simulink model "case3_sensitivity"  (Simulink 6.6)
settings: Solver=ode45  StartTime=0.0  StopTime=36  RelTol=1e-3
undefined symbols (not defined in the file or in its folder): sigbuilder_block
settings Model: Creator=MXKana  LastModifiedBy=mxkana

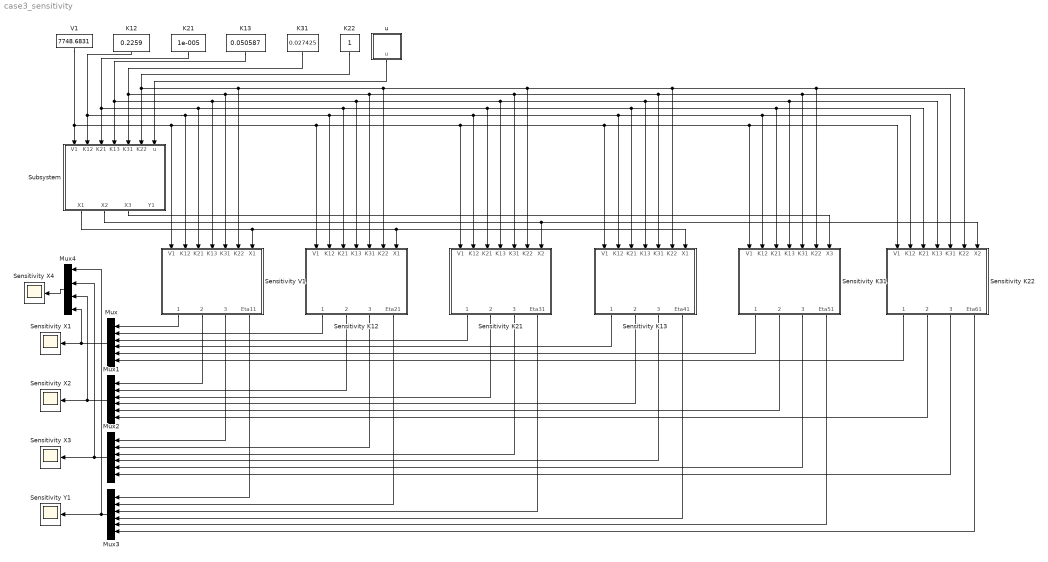
== system case3_sensitivity ==
  K12 : Constant  Orientation=down  Value=0.2259
  K13 : Constant  Orientation=down  Value=0.050587
  K21 : Constant  Orientation=down  Value=1e-005
  K22 : Constant  Orientation=down
  K31 : Constant  Orientation=down  Value=0.027425
  Mux{,1..3} (4 alike) : Mux  Orientation=left  Inputs=6
  Mux4 : Mux  Orientation=left
  Sensitivity K12 : Subsystem  Orientation=down
  Sensitivity K13 : Subsystem  Orientation=down
  Sensitivity K21 : Subsystem  Orientation=down
  Sensitivity K22 : Subsystem  Orientation=down
  Sensitivity K31 : Subsystem  Orientation=down
  Sensitivity V1 : Subsystem  Orientation=down
  Sensitivity X{1..4} (4 alike) : Scope
      Sensitivity X3 settings: SaveName=ScopeData2
      Sensitivity X4 settings: SaveName=ScopeData4
  Sensitivity Y1 : Scope
      settings: SaveName=ScopeData5
  Subsystem : Subsystem  Orientation=down
  V1 : Constant  Orientation=down  Value=7748.6831
  u : Subsystem  Tag=STV Subsys  Orientation=down  LoadFcn=sigbuilder_block('load');  StartFcn=sigbuilder_block('start');  StopFcn=sigbuilder_block('stop');  ClipboardFcn=sigbuilder_block('clipboard');  mask(Sigbuilder block){}
      mask help: Sigbuilder GUI
      mask init:
      | if ~strcmp(get_param(bdroot(gcbh),'SimulationStatus'),'stopped') tuvar = sigbuilder_block('maskInit'); end
      settings: CopyFcn=sigbuilder_block('copy');  DeleteFcn=sigbuilder_block('delete');  ModelCloseFcn=sigbuilder_block('modelClose');  PreSaveFcn=sigbuilder_block('preSave');  NameChangeFcn=sigbuilder_block('namechange');  OpenFcn=sigbuilder_block('open',[406.5 183 550.5 363.75 ]);  CloseFcn=sigbuilder_block('close');
      mask Display: plot(0,0,100,100,[10,10,40,40,10],[80,20,20,80,80],[40,10],[50,50], [40,27,10],[65,72,56],[40,25,25,10],[28,28,43,43]);
  wires:
  V1/1 -> Subsystem/1(V1), Sensitivity V1/1(V1), Sensitivity K12/1(V1), Sensitivity K21/1(V1), Sensitivity K13/1(V1), Sensitivity K31/1(V1), Sensitivity K22/1(V1)
  K12/1 -> Subsystem/2(K12), Sensitivity V1/2(K12), Sensitivity K12/2(K12), Sensitivity K21/2(K12), Sensitivity K13/2(K12), Sensitivity K31/2(K12), Sensitivity K22/2(K12)
  K21/1 -> Subsystem/3(K21), Sensitivity V1/3(K21), Sensitivity K12/3(K21), Sensitivity K21/3(K21), Sensitivity K13/3(K21), Sensitivity K31/3(K21), Sensitivity K22/3(K21)
  K13/1 -> Subsystem/4(K13), Sensitivity V1/4(K13), Sensitivity K12/4(K13), Sensitivity K21/4(K13), Sensitivity K13/4(K13), Sensitivity K31/4(K13), Sensitivity K22/4(K13)
  K31/1 -> Subsystem/5(K31), Sensitivity V1/5(K31), Sensitivity K12/5(K31), Sensitivity K21/5(K31), Sensitivity K13/5(K31), Sensitivity K31/5(K31), Sensitivity K22/5(K31)
  K22/1 -> Subsystem/6(K22), Sensitivity V1/6(K22), Sensitivity K12/6(K22), Sensitivity K21/6(K22), Sensitivity K13/6(K22), Sensitivity K31/6(K22), Sensitivity K22/6(K22)
  u/1(u) -> Subsystem/7(u)
  Subsystem/1(X1) -> Sensitivity V1/7(X1), Sensitivity K12/7(X1), Sensitivity K13/7(X1)
  Subsystem/2(X2) -> Sensitivity K21/7(X2), Sensitivity K22/7(X2)
  Subsystem/3(X3) -> Sensitivity K31/7(X3)
  Sensitivity V1/1(Lambda11) -> Mux/1
  Sensitivity K12/1(Lambda21) -> Mux/2
  Sensitivity K21/1(Lambda31) -> Mux/3
  Sensitivity K13/1(Lambda41) -> Mux/4
  Sensitivity K31/1(Lambda51) -> Mux/5
  Sensitivity K22/1(Lambda61) -> Mux/6
  Mux/1 -> Sensitivity X1/1, Mux4/4
  Mux1/1 -> Sensitivity X2/1, Mux4/3
  Sensitivity V1/2(Lambda12) -> Mux1/1
  Sensitivity K12/2(Lambda22) -> Mux1/2
  Sensitivity K21/2(Lambda32) -> Mux1/3
  Sensitivity K13/2(Lambda42) -> Mux1/4
  Sensitivity K31/2(Lambda52) -> Mux1/5
  Sensitivity K22/2(Lambda62) -> Mux1/6
  Mux2/1 -> Sensitivity X3/1, Mux4/2
  Sensitivity V1/3(Lambda13) -> Mux2/1
  Sensitivity K12/3(Lambda23) -> Mux2/2
  Sensitivity K21/3(Lambda33) -> Mux2/3
  Sensitivity K13/3(Lambda43) -> Mux2/4
  Sensitivity K31/3(Lambda53) -> Mux2/5
  Sensitivity K22/3(Lambda63) -> Mux2/6
  Mux3/1 -> Mux4/1, Sensitivity Y1/1
  Sensitivity V1/4(Eta11) -> Mux3/1
  Sensitivity K12/4(Eta21) -> Mux3/2
  Sensitivity K21/4(Eta31) -> Mux3/3
  Sensitivity K13/4(Eta41) -> Mux3/4
  Sensitivity K31/4(Eta51) -> Mux3/5
  Sensitivity K22/4(Eta61) -> Mux3/6
  Mux4/1 -> Sensitivity X4/1

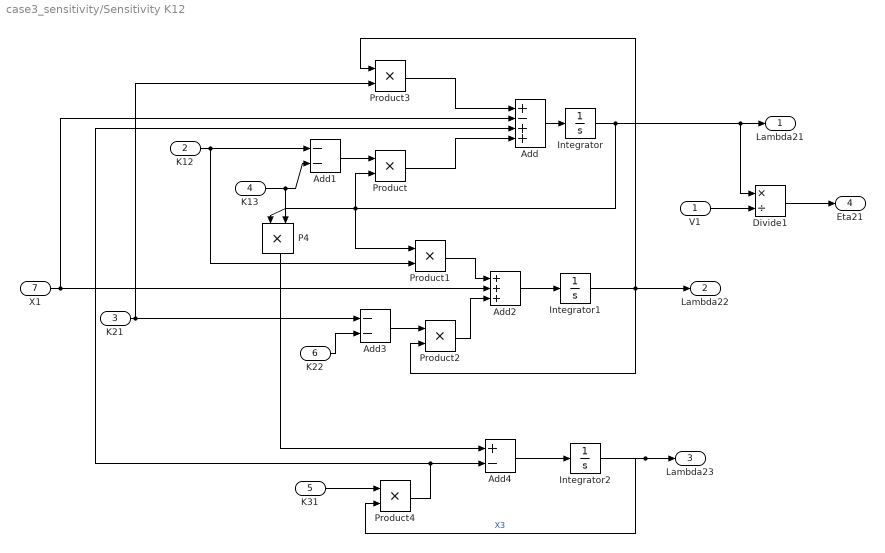
== system case3_sensitivity/Sensitivity K12 ==
  V1 : Inport
  K12 : Inport  Port=2
  K21 : Inport  Port=3
  K13 : Inport  Port=4
  K31 : Inport  Port=5
  K22 : Inport  Port=6
  X1 : Inport  Port=7
  Add : Sum  Inputs=+-++  OutScaling=2^-10
  Add1 : Sum  Inputs=--  OutScaling=2^-10
  Add2 : Sum  Inputs=+++  OutScaling=2^-10
  Add3 : Sum  Inputs=--  OutScaling=2^-10
  Add4 : Sum  Inputs=+-  OutScaling=2^-10
  Divide1 : Product  Inputs=*/  OutScaling=2^-10
  Integrator : Integrator
  Integrator1 : Integrator
  Integrator2 : Integrator
  P4 : Product  Orientation=down  RndMeth=Zero
  Product{,1..4} (5 alike) : Product  RndMeth=Zero
  Lambda21 : Outport
  Lambda22 : Outport  Port=2
  Lambda23 : Outport  Port=3
  Eta21 : Outport  Port=4
  wires:
  Add/1 -> Integrator/1
  K12/1 -> Add1/1, Product1/2
  K13/1 -> Add1/2, P4/1
  Integrator/1 -> Product1/1, Product/2, P4/2, Lambda21/1, Divide1/1
  Add2/1 -> Integrator1/1
  Product1/1 -> Add2/1
  K21/1 -> Add3/1, Product3/2
  K22/1 -> Add3/2
  Add3/1 -> Product2/1
  Integrator1/1 -> Product2/2, Product3/1, Lambda22/1
  Add1/1 -> Product/1
  Add4/1 -> Integrator2/1
  K31/1 -> Product4/1
  P4/1 -> Add4/1
  Product4/1 -> Add4/2, Add/3
  Integrator2/1 -> Product4/2, Lambda23/1  "X3"
  Product3/1 -> Add/1
  V1/1 -> Divide1/2
  X1/1 -> Add/2, Add2/2
  Divide1/1 -> Eta21/1
  Product/1 -> Add/4
  Product2/1 -> Add2/3

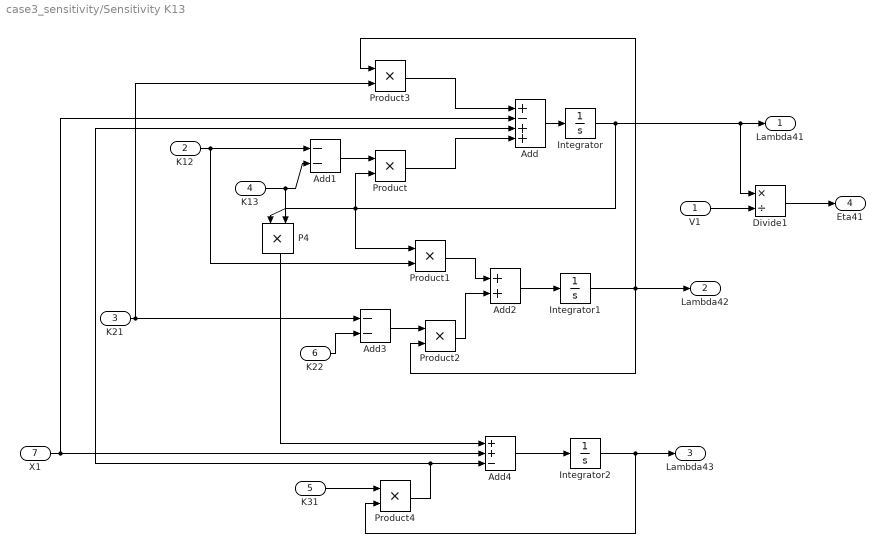
== system case3_sensitivity/Sensitivity K13 ==
  V1 : Inport
  K12 : Inport  Port=2
  K21 : Inport  Port=3
  K13 : Inport  Port=4
  K31 : Inport  Port=5
  K22 : Inport  Port=6
  X1 : Inport  Port=7
  Add : Sum  Inputs=+-++  OutScaling=2^-10
  Add1 : Sum  Inputs=--  OutScaling=2^-10
  Add2 : Sum  OutScaling=2^-10
  Add3 : Sum  Inputs=--  OutScaling=2^-10
  Add4 : Sum  Inputs=++-  OutScaling=2^-10
  Divide1 : Product  Inputs=*/  OutScaling=2^-10
  Integrator : Integrator
  Integrator1 : Integrator
  Integrator2 : Integrator
  P4 : Product  Orientation=down  RndMeth=Zero
  Product{,1..4} (5 alike) : Product  RndMeth=Zero
  Lambda41 : Outport
  Lambda42 : Outport  Port=2
  Lambda43 : Outport  Port=3
  Eta41 : Outport  Port=4
  wires:
  Add/1 -> Integrator/1
  K12/1 -> Add1/1, Product1/2
  K13/1 -> Add1/2, P4/1
  Integrator/1 -> Product1/1, Product/2, P4/2, Lambda41/1, Divide1/1
  Add2/1 -> Integrator1/1
  Product1/1 -> Add2/1
  K21/1 -> Add3/1, Product3/2
  K22/1 -> Add3/2
  Add3/1 -> Product2/1
  Integrator1/1 -> Product2/2, Product3/1, Lambda42/1
  Add1/1 -> Product/1
  Add4/1 -> Integrator2/1
  K31/1 -> Product4/1
  P4/1 -> Add4/1
  Product4/1 -> Add/3, Add4/3
  Integrator2/1 -> Product4/2, Lambda43/1
  Product3/1 -> Add/1
  V1/1 -> Divide1/2
  X1/1 -> Add/2, Add4/2
  Divide1/1 -> Eta41/1
  Product/1 -> Add/4
  Product2/1 -> Add2/2

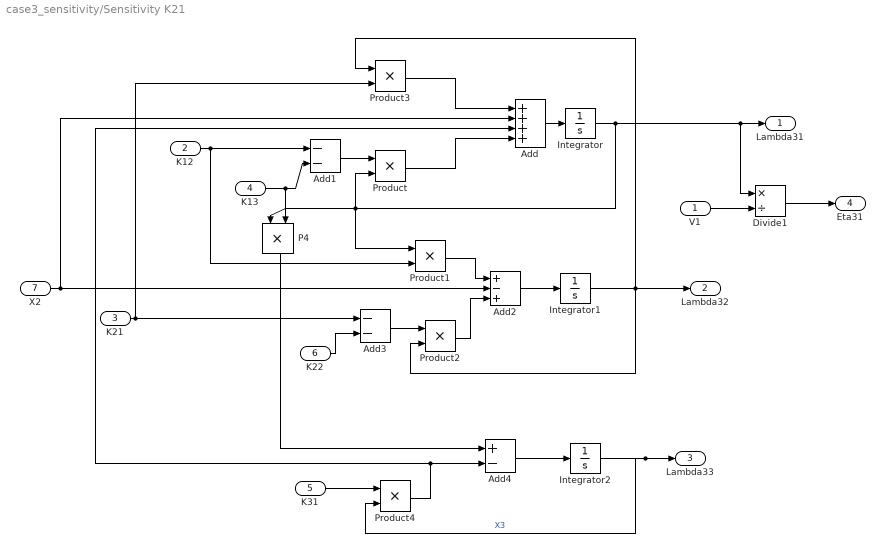
== system case3_sensitivity/Sensitivity K21 ==
  V1 : Inport
  K12 : Inport  Port=2
  K21 : Inport  Port=3
  K13 : Inport  Port=4
  K31 : Inport  Port=5
  K22 : Inport  Port=6
  X2 : Inport  Port=7
  Add : Sum  Inputs=++++  OutScaling=2^-10
  Add1 : Sum  Inputs=--  OutScaling=2^-10
  Add2 : Sum  Inputs=+-+  OutScaling=2^-10
  Add3 : Sum  Inputs=--  OutScaling=2^-10
  Add4 : Sum  Inputs=+-  OutScaling=2^-10
  Divide1 : Product  Inputs=*/  OutScaling=2^-10
  Integrator : Integrator
  Integrator1 : Integrator
  Integrator2 : Integrator
  P4 : Product  Orientation=down  RndMeth=Zero
  Product{,1..4} (5 alike) : Product  RndMeth=Zero
  Lambda31 : Outport
  Lambda32 : Outport  Port=2
  Lambda33 : Outport  Port=3
  Eta31 : Outport  Port=4
  wires:
  Add/1 -> Integrator/1
  K12/1 -> Add1/1, Product1/2
  K13/1 -> Add1/2, P4/1
  Integrator/1 -> Product1/1, Product/2, P4/2, Lambda31/1, Divide1/1
  Add2/1 -> Integrator1/1
  Product1/1 -> Add2/1
  K21/1 -> Add3/1, Product3/2
  K22/1 -> Add3/2
  Add3/1 -> Product2/1
  Integrator1/1 -> Product2/2, Product3/1, Lambda32/1
  Add1/1 -> Product/1
  Add4/1 -> Integrator2/1
  K31/1 -> Product4/1
  P4/1 -> Add4/1
  Product4/1 -> Add4/2, Add/3
  Integrator2/1 -> Product4/2, Lambda33/1  "X3"
  Product3/1 -> Add/1
  V1/1 -> Divide1/2
  X2/1 -> Add/2, Add2/2
  Divide1/1 -> Eta31/1
  Product/1 -> Add/4
  Product2/1 -> Add2/3

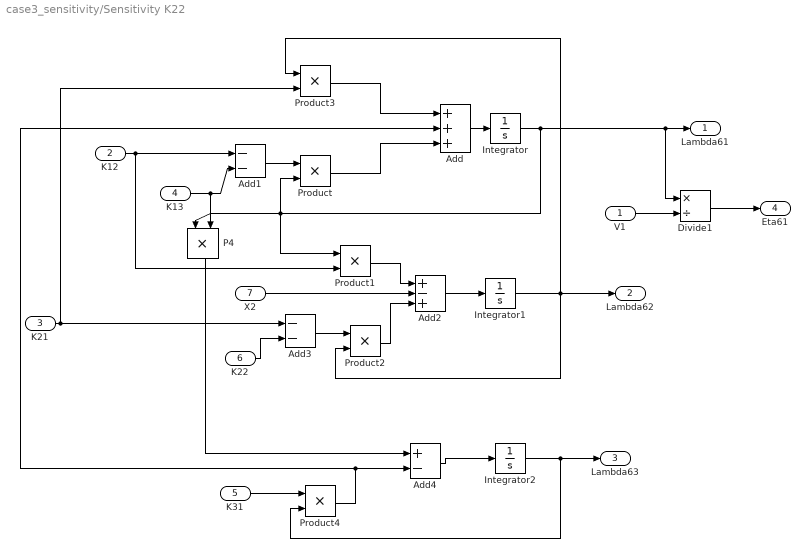
== system case3_sensitivity/Sensitivity K22 ==
  V1 : Inport
  K12 : Inport  Port=2
  K21 : Inport  Port=3
  K13 : Inport  Port=4
  K31 : Inport  Port=5
  K22 : Inport  Port=6
  X2 : Inport  Port=7
  Add : Sum  Inputs=+++  OutScaling=2^-10
  Add1 : Sum  Inputs=--  OutScaling=2^-10
  Add2 : Sum  Inputs=+-+  OutScaling=2^-10
  Add3 : Sum  Inputs=--  OutScaling=2^-10
  Add4 : Sum  Inputs=+-  OutScaling=2^-10
  Divide1 : Product  Inputs=*/  OutScaling=2^-10
  Integrator : Integrator
  Integrator1 : Integrator
  Integrator2 : Integrator
  P4 : Product  Orientation=down  RndMeth=Zero
  Product{,1..4} (5 alike) : Product  RndMeth=Zero
  Lambda61 : Outport
  Lambda62 : Outport  Port=2
  Lambda63 : Outport  Port=3
  Eta61 : Outport  Port=4
  wires:
  Add/1 -> Integrator/1
  K12/1 -> Add1/1, Product1/2
  K13/1 -> Add1/2, P4/1
  Integrator/1 -> Product1/1, Product/2, P4/2, Lambda61/1, Divide1/1
  Add2/1 -> Integrator1/1
  Product1/1 -> Add2/1
  K21/1 -> Add3/1, Product3/2
  K22/1 -> Add3/2
  Add3/1 -> Product2/1
  Integrator1/1 -> Product2/2, Product3/1, Lambda62/1
  Add1/1 -> Product/1
  Add4/1 -> Integrator2/1
  K31/1 -> Product4/1
  P4/1 -> Add4/1
  Product4/1 -> Add4/2, Add/2
  Integrator2/1 -> Product4/2, Lambda63/1
  Product3/1 -> Add/1
  V1/1 -> Divide1/2
  Divide1/1 -> Eta61/1
  Product/1 -> Add/3
  Product2/1 -> Add2/3
  X2/1 -> Add2/2

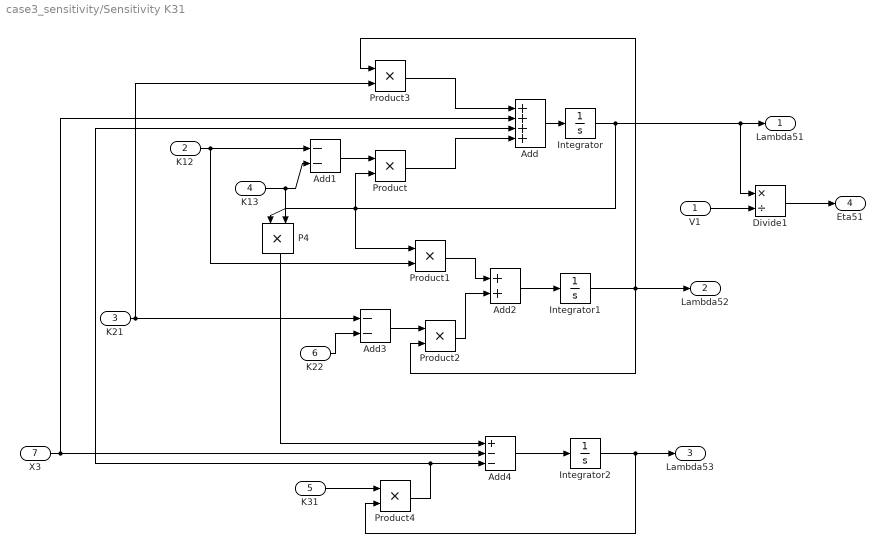
== system case3_sensitivity/Sensitivity K31 ==
  V1 : Inport
  K12 : Inport  Port=2
  K21 : Inport  Port=3
  K13 : Inport  Port=4
  K31 : Inport  Port=5
  K22 : Inport  Port=6
  X3 : Inport  Port=7
  Add : Sum  Inputs=++++  OutScaling=2^-10
  Add1 : Sum  Inputs=--  OutScaling=2^-10
  Add2 : Sum  OutScaling=2^-10
  Add3 : Sum  Inputs=--  OutScaling=2^-10
  Add4 : Sum  Inputs=+--  OutScaling=2^-10
  Divide1 : Product  Inputs=*/  OutScaling=2^-10
  Integrator : Integrator
  Integrator1 : Integrator
  Integrator2 : Integrator
  P4 : Product  Orientation=down  RndMeth=Zero
  Product{,1..4} (5 alike) : Product  RndMeth=Zero
  Lambda51 : Outport
  Lambda52 : Outport  Port=2
  Lambda53 : Outport  Port=3
  Eta51 : Outport  Port=4
  wires:
  Add/1 -> Integrator/1
  K12/1 -> Add1/1, Product1/2
  K13/1 -> Add1/2, P4/1
  Integrator/1 -> Product1/1, Product/2, P4/2, Lambda51/1, Divide1/1
  Add2/1 -> Integrator1/1
  Product1/1 -> Add2/1
  K21/1 -> Add3/1, Product3/2
  K22/1 -> Add3/2
  Add3/1 -> Product2/1
  Integrator1/1 -> Product2/2, Product3/1, Lambda52/1
  Add1/1 -> Product/1
  Add4/1 -> Integrator2/1
  K31/1 -> Product4/1
  P4/1 -> Add4/1
  Product4/1 -> Add/3, Add4/3
  Integrator2/1 -> Product4/2, Lambda53/1
  Product3/1 -> Add/1
  V1/1 -> Divide1/2
  X3/1 -> Add/2, Add4/2
  Divide1/1 -> Eta51/1
  Product/1 -> Add/4
  Product2/1 -> Add2/2

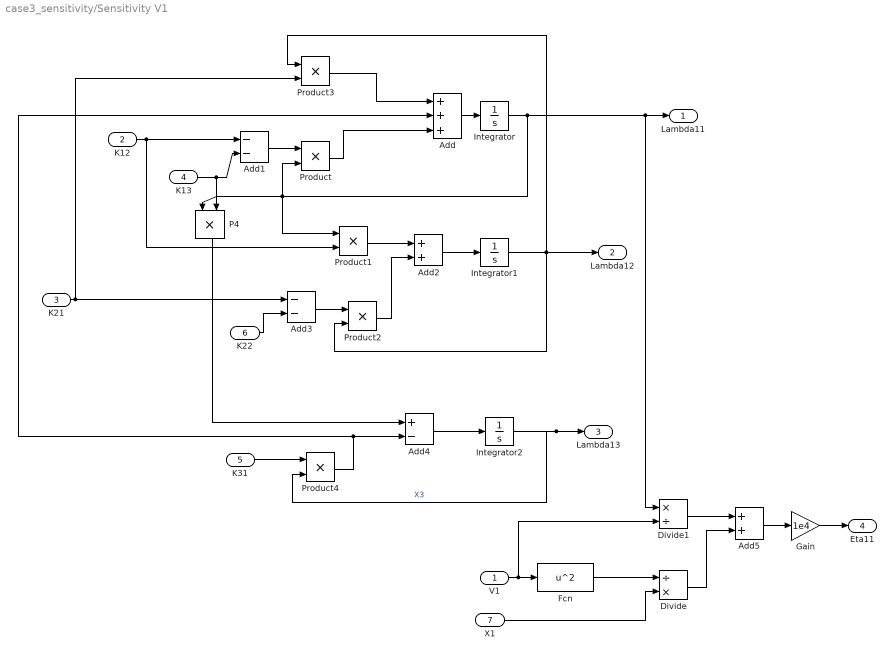
== system case3_sensitivity/Sensitivity V1 ==
  V1 : Inport
  K12 : Inport  Port=2
  K21 : Inport  Port=3
  K13 : Inport  Port=4
  K31 : Inport  Port=5
  K22 : Inport  Port=6
  X1 : Inport  Port=7
  Add : Sum  Inputs=+++  OutScaling=2^-10
  Add1 : Sum  Inputs=--  OutScaling=2^-10
  Add2 : Sum  OutScaling=2^-10
  Add3 : Sum  Inputs=--  OutScaling=2^-10
  Add4 : Sum  Inputs=+-  OutScaling=2^-10
  Add5 : Sum  OutScaling=2^-10
  Divide : Product  Inputs=/*  OutScaling=2^-10
  Divide1 : Product  Inputs=*/  OutScaling=2^-10
  Fcn : Fcn  Expr=u^2
  Gain : Gain  Gain=1e4
  Integrator : Integrator
  Integrator1 : Integrator
  Integrator2 : Integrator
  P4 : Product  Orientation=down  RndMeth=Zero
  Product{,1..4} (5 alike) : Product  RndMeth=Zero
  Lambda11 : Outport
  Lambda12 : Outport  Port=2
  Lambda13 : Outport  Port=3
  Eta11 : Outport  Port=4
  wires:
  Add/1 -> Integrator/1
  K12/1 -> Add1/1, Product1/2
  K13/1 -> Add1/2, P4/1
  Integrator/1 -> Product1/1, Product/2, P4/2, Lambda11/1, Divide1/1
  Add2/1 -> Integrator1/1
  Product1/1 -> Add2/1
  K21/1 -> Add3/1, Product3/2
  K22/1 -> Add3/2
  Add3/1 -> Product2/1
  Integrator1/1 -> Product2/2, Product3/1, Lambda12/1
  Product2/1 -> Add2/2
  Add1/1 -> Product/1
  Product/1 -> Add/3
  Add4/1 -> Integrator2/1
  K31/1 -> Product4/1
  P4/1 -> Add4/1
  Product4/1 -> Add4/2, Add/2
  Integrator2/1 -> Product4/2, Lambda13/1  "X3"
  Product3/1 -> Add/1
  V1/1 -> Fcn/1, Divide1/2
  X1/1 -> Divide/2
  Fcn/1 -> Divide/1
  Divide/1 -> Add5/2
  Divide1/1 -> Add5/1
  Add5/1 -> Gain/1
  Gain/1 -> Eta11/1

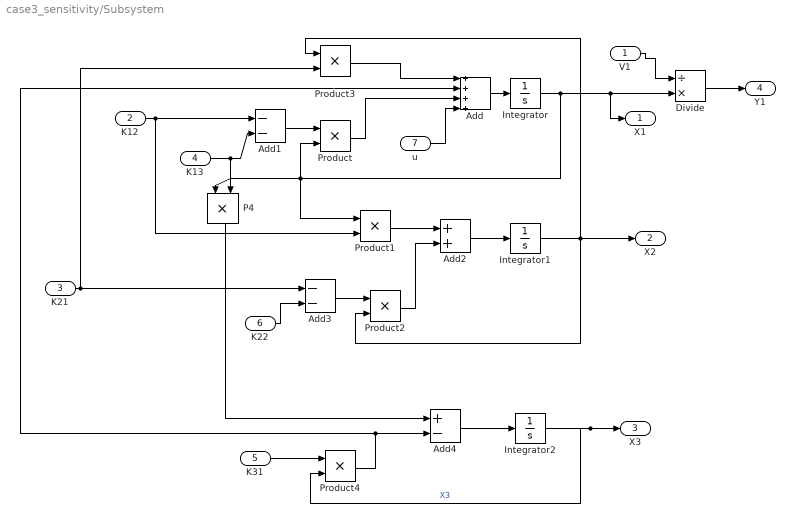
== system case3_sensitivity/Subsystem ==
  V1 : Inport
  K12 : Inport  Port=2
  K21 : Inport  Port=3
  K13 : Inport  Port=4
  K31 : Inport  Port=5
  K22 : Inport  Port=6
  u : Inport  Port=7
  Add : Sum  Inputs=++++  OutScaling=2^-10
  Add1 : Sum  Inputs=--  OutScaling=2^-10
  Add2 : Sum  OutScaling=2^-10
  Add3 : Sum  Inputs=--  OutScaling=2^-10
  Add4 : Sum  Inputs=+-  OutScaling=2^-10
  Divide : Product  Inputs=/*  OutScaling=2^-10
  Integrator : Integrator
  Integrator1 : Integrator
  Integrator2 : Integrator
  P4 : Product  Orientation=down  RndMeth=Zero
  Product{,1..4} (5 alike) : Product  RndMeth=Zero
  X1 : Outport
  X2 : Outport  Port=2
  X3 : Outport  Port=3
  Y1 : Outport  Port=4
  wires:
  Add/1 -> Integrator/1
  K12/1 -> Add1/1, Product1/2
  K13/1 -> Add1/2, P4/1
  Integrator/1 -> Product1/1, Product/2, P4/2, Divide/2, X1/1
  Add2/1 -> Integrator1/1
  Product1/1 -> Add2/1
  K21/1 -> Add3/1, Product3/2
  K22/1 -> Add3/2
  Add3/1 -> Product2/1
  Integrator1/1 -> Product2/2, Product3/1, X2/1
  Product2/1 -> Add2/2
  Add1/1 -> Product/1
  Product/1 -> Add/3
  Add4/1 -> Integrator2/1
  K31/1 -> Product4/1
  P4/1 -> Add4/1
  Product4/1 -> Add4/2, Add/2
  Integrator2/1 -> Product4/2, X3/1  "X3"
  Product3/1 -> Add/1
  u/1 -> Add/4
  V1/1 -> Divide/1
  Divide/1 -> Y1/1

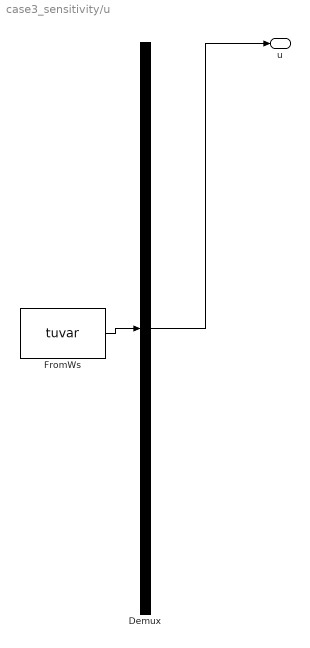
== system case3_sensitivity/u ==
  Demux : Demux  Tag=STV Demux  Outputs=1
  FromWs : FromWorkspace  Tag=STV FromWs  VariableName=tuvar  SampleTime=0  SigBuilderData=DataTag0  VnvData=DataTag1
      SigBuilderData=|
      | channels.label = 'u'
      | channels.allXData = {[0 1 1 36]}
      | channels.allYData = {[100000 100000 0 0]}
      | common.afterFinalStr = 'Extrapolate'
      | common.sampleTime = 0
      | dataSet.timeRange = [0 36]
      | dataSet.name = 'Group 1'
  u : Outport  Tag=STV Outport
  wires:
  Demux/1 -> u/1
  FromWs/1 -> Demux/1
